simulink model "pid_sim"  (R2021a)
settings: Solver=FixedStepAuto  StartTime=0.0  StopTime=1000  FixedStep=1  RelTol=1e-3
values from neighbouring files (symbols this model uses):
  delay = 10    [pid_controller_config.m]
  dt = 1    [pid_controller_config.m]    (also in pid_controller_plot_results.m)
  k = 8.65/input_amplitude    (= 9.61111111111)    [pid_controller_config.m]
  kd = 0    [pid_controller_config.m]
  ki = 0.0039    [pid_controller_config.m]
  kp = 0.93    [pid_controller_config.m]
  system_offset = 22.95    [pid_controller_config.m]
  T = 300    [pid_controller_config.m]
libraries: pid_lib x1
settings Model: Creator=dawidexpompa2000  LastModifiedBy=dawidexpompa2000

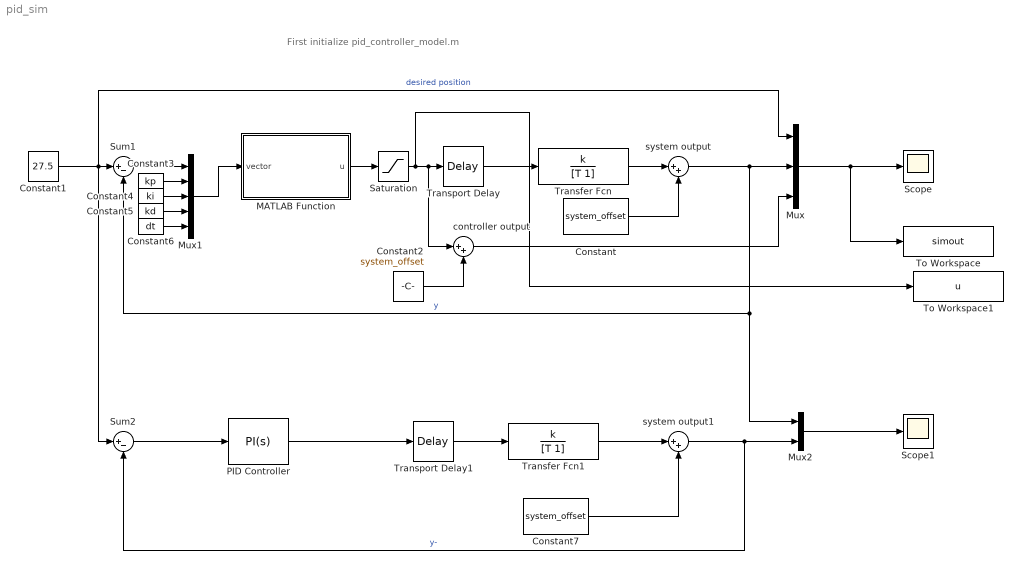
== system pid_sim ==
  note: First initialize pid_controller_model.m
  Constant : Constant  Value=system_offset
  Constant1 : Constant  Value=27.5
  Constant2 : Constant  Value=system_offset
  Constant3 : Constant  Value=kp
  Constant4 : Constant  Value=ki
  Constant5 : Constant  Value=kd
  Constant6 : Constant  Value=dt
  Constant7 : Constant  Value=system_offset
  MATLAB Function : MATLAB Function  TreatAsAtomicUnit=on
  Mux : Mux  Inputs=3
  Mux1 : Mux  Inputs=5
  Mux2 : Mux  Inputs=2
  PID Controller : pid_lib/PID Controller  Controller=PI  Form=Parallel  TimeDomain=Continuous-time  UseExternalTs=off  SampleTime=-1  IntegratorMethod=Forward Euler  FilterMethod=Forward Euler  ControllerParametersSource=internal  P=0.607338773069937  I=0.00245637321622817  D=0  UseFilter=on  N=100  TunerSelectOption=Transfer Function Based (PID Tuner App)  InitialConditionSource=internal  InitialConditionForIntegrator=0  InitialConditionForFilter=0  DifferentiatorICPrevScaledInput=0  ExternalReset=none  TrackingMode=off  Kt=1  LimitOutput=on  SatLimitsSource=internal  UpperSaturationLimit=1  LowerSaturationLimit=0  LinearizeAsGain=off  AntiWindupMode=none  Kb=1  POutMin=[]  POutMax=[]  IOutMin=[]  IOutMax=[]  DOutMin=[]  DOutMax=[]  NOutMin=[]  NOutMax=[]  SumOutMin=[]  SumOutMax=[]  SaturationOutMin=[]  SaturationOutMax=[]  PParamMin=[]  PParamMax=[]  IParamMin=[]  IParamMax=[]  DParamMin=[]  DParamMax=[]  NParamMin=[]  NParamMax=[]  KbParamMin=[]  KbParamMax=[]  KtParamMin=[]  KtParamMax=[]  KbOutMin=[]  KbOutMax=[]  KtOutMin=[]  KtOutMax=[]  IntegratorOutMin=[]  IntegratorOutMax=[]  FilterOutMin=[]  FilterOutMax=[]  SumI1OutMin=[]  SumI1OutMax=[]  SumI2OutMin=[]  SumI2OutMax=[]  SumI3OutMin=[]  SumI3OutMax=[]  SumI4OutMin=[]  SumI4OutMax=[]  SumDOutMin=[]  SumDOutMax=[]  DifferentiatorOutMin=[]  DifferentiatorOutMax=[]  FilterDiffOutCoefMin=[]  FilterDiffOutCoefMax=[]  ReciprocalOutMin=[]  ReciprocalOutMax=[]  SumDenOutMin=[]  SumDenOutMax=[]  SumNumOutMin=[]  SumNumOutMax=[]  DivideOutMin=[]  DivideOutMax=[]  UdiffTsProdOutMin=[]  UdiffTsProdOutMax=[]  NTsProdOutMin=[]  NTsProdOutMax=[]  UintegralTsProdOutMin=[]  UintegralTsProdOutMax=[]  UngainTsProdOutMin=[]  UngainTsProdOutMax=[]  IntegratorContinuousStateAttributes=''  IntegratorStateMustResolveToSignalObject=off  IntegratorRTWStateStorageClass=Auto  FilterContinuousStateAttributes=''  FilterStateMustResolveToSignalObject=off  FilterRTWStateStorageClass=Auto  ParallelPVariant=InternalParameters  IdealPVariant=Disabled  IVariant=InternalParameters  DVariant=Disabled  IntegratorVariant=Continuous  SatVariant=Enabled  AWVariant=Passthrough  PCopyVariant=Disabled  TRVariant=Disabled  FdbkBlocksVariant=Forward  IdealPFdbkVariant=Disabled  SatFdbkVariant=Disabled  DerivativeFilterVariant=Disabled  NVariant=Disabled  NCopyVariant=Disabled_SignalSpec  FilterICVariant=Disabled  IntegratorICVariant=InternalICs  ExternalResetVariant=Disabled  TRSumVariant=Passthrough  SumFdbkVariant=Disabled  SumVariant=Sum_PI  TsampFilterVariant=InternalTs  TsampNgainVariant=Passthrough  TsampIntegralVariant=Passthrough  ExternalSaturationOutDataTypeStr=Inherit: Same as second input
  Saturation : Saturate  UpperLimit=1  LowerLimit=0
  Scope : Scope
  Scope1 : Scope
  Sum1 : Sum  Inputs=|+-
  Sum2 : Sum  Inputs=|+-
  To Workspace : ToWorkspace  VariableName=simout  SaveFormat=Timeseries  SampleTime=-1
  To Workspace1 : ToWorkspace  VariableName=u  SaveFormat=Timeseries  SampleTime=-1
  Transfer Fcn : TransferFcn  Numerator=k  Denominator=[T 1]
  Transfer Fcn1 : TransferFcn  Numerator=k  Denominator=[T 1]
  Transport Delay : TransportDelay  DelayTime=delay
  Transport Delay1 : TransportDelay  DelayTime=delay
  controller output : Sum  Inputs=|++
  system output : Sum  Inputs=|++
  system output1 : Sum  Inputs=|++
  wires:
  Transport Delay/1 -> Transfer Fcn/1
  Transfer Fcn/1 -> system output/1
  Constant/1 -> system output/2
  system output/1 -> Mux2/1, Sum1/2, Mux/2  "y"
  Mux/1 -> To Workspace/1, Scope/1
  Constant1/1 -> Sum2/1, Mux/1, Sum1/1  "desired position"
  controller output/1 -> Mux/3
  Constant2/1 -> controller output/2
  Saturation/1 -> To Workspace1/1, controller output/1, Transport Delay/1
  MATLAB Function/1(u) -> Saturation/1
  Mux1/1 -> MATLAB Function/1(vector)
  Sum1/1 -> Mux1/1
  Constant3/1 -> Mux1/2
  Constant4/1 -> Mux1/3
  Constant5/1 -> Mux1/4
  Constant6/1 -> Mux1/5
  PID Controller/1 -> Transport Delay1/1
  Transport Delay1/1 -> Transfer Fcn1/1
  Transfer Fcn1/1 -> system output1/1
  Constant7/1 -> system output1/2
  system output1/1 -> Mux2/2, Sum2/2  "y-"
  Mux2/1 -> Scope1/1
  Sum2/1 -> PID Controller/1

== matlab function pid_sim/MATLAB Function ==
  settings: updateMethod=DISCRETE
  data: vector input; u output
function u = pid_controller(vector)
%separate data from passed vector:
e = vector(1);
kp = vector(2);
ki = vector(3);
kd = vector(4);
dt = vector(5);

%static value
persistent previous_error;
if isempty(previous_error)
    previous_error = 0;
end

persistent previous_integral;
if isempty(previous_integral)
    previous_integral = 0;
end

%controller equations:
%%proprotional part
P = kp*e;

%%integral part
integral = previous_integral + (e+previous_error) ; %numerical integrator without anti-windup
previous_integral = integral;
I = ki*integral*(dt/2);

%%derivative part
derivative = (e - previous_error)/dt;
previous_error = e;
D = kd*derivative;


u = P + I + D;
